simulink model "gear_with_1_gain"  (R2020b)
settings: Solver=VariableStepAuto  StartTime=0.0  StopTime=10.0  RelTol=1e-3
settings Model: Creator=morro  LastModifiedBy=morro

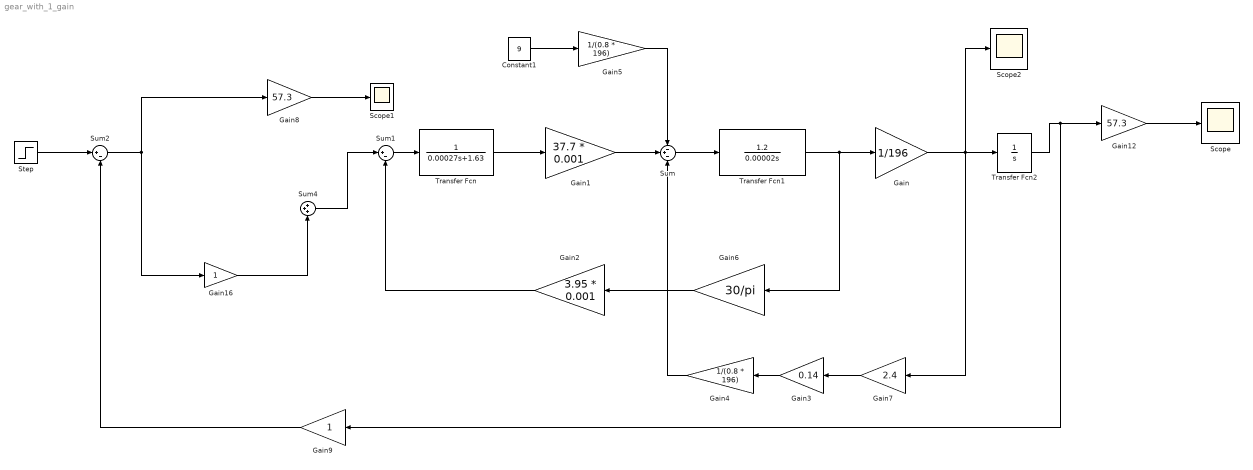
== system gear_with_1_gain ==
  Constant1 : Constant  Value=9
  Gain : Gain  Gain=1/196
  Gain1 : Gain  Gain=37.7 * 0.001
  Gain12 : Gain  Gain=57.3
  Gain16 : Gain
  Gain2 : Gain  Gain=3.95 * 0.001
  Gain3 : Gain  Gain=0.14
  Gain4 : Gain  Gain=1/(0.8 * 196)
  Gain5 : Gain  Gain=1/(0.8 * 196)
  Gain6 : Gain  Gain=30/pi
  Gain7 : Gain  Gain=2.4
  Gain8 : Gain  Gain=57.3
  Gain9 : Gain
  Scope : Scope
  Scope1 : Scope
  Scope2 : Scope
  Step : Step  After=25/57.3  SampleTime=0
  Sum : Sum  Inputs=-+-
  Sum1 : Sum  Inputs=|+-
  Sum2 : Sum  Inputs=|+-
  Sum4 : Sum  Inputs=+++
  Transfer Fcn : TransferFcn  Denominator=[0.00027 1.63]
  Transfer Fcn1 : TransferFcn  Numerator=[1.2]  Denominator=[0.00002 0]
  Transfer Fcn2 : TransferFcn  Denominator=[1 0]
  wires:
  Gain6/1 -> Gain2/1
  Gain12/1 -> Scope/1
  Sum4/1 -> Sum1/1
  Constant1/1 -> Gain5/1
  Gain8/1 -> Scope1/1
  Transfer Fcn1/1 -> Gain6/1, Gain/1
  Gain3/1 -> Gain4/1
  Step/1 -> Sum2/1
  Gain9/1 -> Sum2/2
  Gain5/1 -> Sum/1
  Sum2/1 -> Gain16/1, Gain8/1
  Transfer Fcn/1 -> Gain1/1
  Gain2/1 -> Sum1/2
  Transfer Fcn2/1 -> Gain9/1, Gain12/1
  Gain/1 -> Scope2/1, Gain7/1, Transfer Fcn2/1
  Gain16/1 -> Sum4/3
  Sum1/1 -> Transfer Fcn/1
  Gain4/1 -> Sum/3
  Gain1/1 -> Sum/2
  Sum/1 -> Transfer Fcn1/1
  Gain7/1 -> Gain3/1
